simulink model "experiment"  (R2018a)
settings: Solver=ode4  StartTime=0.0  StopTime=10.0  FixedStep=1e-2  RelTol=1e-3
values from neighbouring files (symbols this model uses):
  bot = botl(f,:)    [MarcinGrzybS.m]
  top = topl(f,:)    [MarcinGrzybS.m]
settings Model: Creator=nicra  LastModifiedBy=nicra

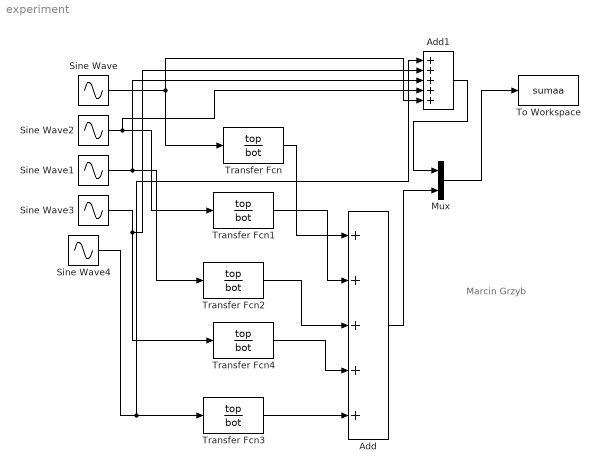
== system experiment ==
  note: Marcin Grzyb
  Add : Sum  Inputs=+++++
  Add1 : Sum  Inputs=+++++
  Mux : Mux  Inputs=2
  Sine Wave : Sin  Amplitude=2  Frequency=0.001  Phase=1  SampleTime=0
  Sine Wave1 : Sin  Frequency=30  Phase=2  SampleTime=0
  Sine Wave2 : Sin  Amplitude=3  Phase=5  SampleTime=0
  Sine Wave3 : Sin  Amplitude=2  Frequency=0.01  Phase=1  SampleTime=0
  Sine Wave4 : Sin  Amplitude=4  Frequency=5  SampleTime=0
  To Workspace : ToWorkspace  VariableName=sumaa  SaveFormat=Timeseries  SampleTime=-1
  Transfer Fcn{,1..4} (5 alike) : TransferFcn  Numerator=top  Denominator=bot
  wires:
  Sine Wave/1 -> Add1/5, Transfer Fcn/1
  Sine Wave2/1 -> Add1/4, Transfer Fcn1/1
  Sine Wave1/1 -> Add1/3, Transfer Fcn2/1
  Sine Wave3/1 -> Add1/2, Transfer Fcn4/1
  Sine Wave4/1 -> Add1/1, Transfer Fcn3/1
  Transfer Fcn/1 -> Add/1
  Transfer Fcn1/1 -> Add/2
  Transfer Fcn2/1 -> Add/3
  Transfer Fcn4/1 -> Add/4
  Transfer Fcn3/1 -> Add/5
  Add/1 -> Mux/2
  Mux/1 -> To Workspace/1
  Add1/1 -> Mux/1
